simulink model "host_udpcam_demo"  (Simulink 7.3)
settings: Solver=ode45  StartTime=0.0  StopTime=10  RelTol=1e-3
undefined symbols (not defined in the file): gray
libraries: vipsnks x2, waijung_image_sensor_lib x1
settings Model: Creator=Krisada  LastModifiedBy=Krisada

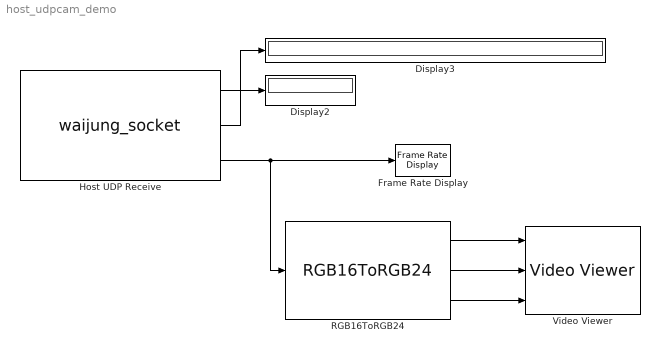
== system host_udpcam_demo ==
  Display2 : Display
  Display3 : Display
  Frame Rate Display : vipsnks/Frame Rate Display  DialogController=vipDDGCreate  DialogControllerArgs=DataTag0  UpdateRate=10
  Host UDP Receive : S-Function  FunctionName=waijung_socket  Parameters=conf,inputporttype,inputportwidth,outputporttype,outputportwidth,address,port,optionstring,sampletime,blockid,options  EnableBusSupport=off  mask(waijung_socket){conf=HostReceive, protocol=UDP, port=7, netadapter=Intel(R) 82579LM Gigabit Network Connection, address=0.0.0.0, echo=off, transfer=Blocking, timeout=5, datasource=BufferStream, datatype=uint16, datacount=120*160, porttype_double=0, porttype_single=0, porttype_int8=0, porttype_uint8=0, porttype_int16=0, porttype_uint16=0, porttype_int32=0, porttype_uint32=1, portpinstr=0, sampletime=0.0001, blockid=HostUDPReceive, inputporttype=[], inputportwidth=[], inputportlabel={}, outputporttype=[5,3,5], outputportwidth=[1,4,19200], outputportlabel={'Remote Port','Remote IP(1:4)','Data(1:19200)'}, compat=0, optionstring=[], options=[7,2,1,5000,1]}
      mask prompts: conf "Configuration"; netadapter "Host Network Adapter"; echo "Echo (Return the receiving data back to sender)"; timeout "Timeout (Seconds)"; datasource "Data"; datatype "Data type"; datacount "Port width"; porttype_double "Number of data port, type DOUBLE"; porttype_single "Number of data port, type SINGLE"; porttype_int8 "Number of data port, type INT8"; porttype_uint8 "Number of data port, type UINT8"; porttype_int16 "Number of data port, type INT16"; porttype_uint16 "Number of data port, type UINT16"; porttype_int32 "Number of data port, type INT32"; porttype_uint32 "Number of data port, type UINT32"; portpinstr "Port Pin String"; sampletime "Sample time (sec)"; blockid "Block ID"; inputporttype "Input Port Type"; inputportwidth "Input Port Width"; inputportlabel "Input Port Label"; outputporttype "Output Port Type"; outputportwidth "Output Port Width"; outputportlabel "Output port label"; compat "Compatibility (Reserved for future use)"; optionstring "String(s) to be passed to TLC"; options "Sim options"
      mask help:
      | Port:
      |  - Port number to open for data receive.
      | Transfer:
      |  - Blocking: CPU is blocked durring wait for data.
      | Timeout:
      |  - Timeout in seconds for wait for data.
      mask init:
      | waijung_socket_callback('init');
      mask Help: web(fullfile(waijungdocroot,'waijung_socket_host_udp_receive.htm'), '-browser')
      mask StyleString: popup(HostSend|HostReceive|TargetSend|TargetReceive),popup(TCP|UDP),edit,popup(Intel(R) 82579LM Gigabit Network Connection),edit,checkbox,popup(Blocking|Non-blocking),edit,popup(Ports|Vector|BufferStream),popup(double|single|int8|uint8|int16|uint16|int32|uint32),edit,edit,edit,edit,edit,edit,edit,edit,edit,edit,edit,edit,edit,edit,edit,edit,edit,edit,edit,edit,edit
      mask CallbackString: waijung_socket_callback('conf');|||waijung_socket_callback('netadapter');|||||waijung_socket_callback('datasource');|||waijung_socket_callback('datatype');|waijung_socket_callback('datatype');|waijung_socket_callback('datatype');|waijung_socket_callback('datatype');|waijung_socket_callback('datatype');|waijung_socket_callback('datatype');|waijung_socket_callback('datatype');|waijung_socket_callback('datatype');||waijung_socket_callback('sampletime');|waijung_socket_callback('blockid');|||||||||
      mask Display: text(0.05, 0.5, '[Host UDP Receive]\nPort: 7\nTs (sec): 0.0001','ver','middle','hor','left'); port_label('output', 1,'Remote Port'); port_label('output', 2,'Remote IP(1:4)'); port_label('output', 3,'Data(1:19200)');
  RGB16ToRGB24 : waijung_image_sensor_lib/RGB16ToRGB24  conf=RGB16ToRGB24  column=120  row=160  inputalignment=RGB  outputalignment=BGR  colorseparate=on  simparams=[0 160 0 1]  portpinstr=0  sampletime=-1  blockid=RGB16ToRGB24  inputporttype=[5]  inputportwidth=[19200]  inputportlabel={'Input'}  outputporttype="[3  3 3]"  outputportwidth=[120 120 120]  outputportlabel={'B','G','R'}  compat=0  optionstring=[]
  Video Viewer : vipsnks/Video Viewer  DialogControllerArgs=DataTag2  inputType=Obsolete7b  imagePorts=Separate color signals  useColorMap=off  colormapValue=gray(256)  specRange=off  minInputVal=0  maxInputVal=255  FigPos=[428 938 475 382]  AxisZoom=on  trueSizedOnce=off  OpenAtMdlStart=on
  wires:
  Host UDP Receive/3 -> RGB16ToRGB24/1, Frame Rate Display/1
  Host UDP Receive/1 -> Display2/1
  Host UDP Receive/2 -> Display3/1
  RGB16ToRGB24/2 -> Video Viewer/2
  RGB16ToRGB24/3 -> Video Viewer/3
  RGB16ToRGB24/1 -> Video Viewer/1
